simulink library "solar_panel_power_lib"  (R2016b)
settings: Solver=VariableStepAuto  StartTime=0.0  StopTime=10.0  RelTol=1e-3
undefined symbols (not defined in the file or in its folder): sim_params
libraries: aerolibutil x1
settings Model: Creator=taylorreynolds  LastModifiedBy=Taylor

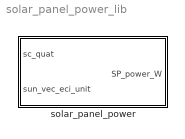
== system solar_panel_power_lib ==
  solar_panel_power : Subsystem

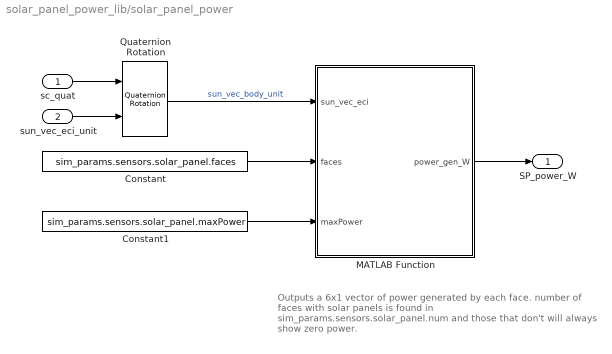
== system solar_panel_power_lib/solar_panel_power ==
  note: Outputs a 6x1 vector of power generated by each face.
      | number of faces with solar panels is found in
      | sim_params.sensors.solar_panel.num
      | and those that don't will always show zero power.
  sc_quat : Inport
  sun_vec_eci_unit : Inport  Port=2
  Constant : Constant  Value=sim_params.sensors.solar_panel.faces
  Constant1 : Constant  Value=sim_params.sensors.solar_panel.maxPower
  MATLAB Function : MATLAB Function  TreatAsAtomicUnit=on
  Quaternion Rotation : aerolibutil/Quaternion Rotation
  SP_power_W : Outport
  wires:
  sun_vec_eci_unit/1 -> Quaternion Rotation/2
  sc_quat/1 -> Quaternion Rotation/1
  MATLAB Function/1(power_gen_W) -> SP_power_W/1
  Quaternion Rotation/1 -> MATLAB Function/1(sun_vec_eci)  "sun_vec_body_unit"
  Constant/1 -> MATLAB Function/2(faces)
  Constant1/1 -> MATLAB Function/3(maxPower)

== matlab function solar_panel_power_lib/solar_panel_power/MATLAB Function ==
  data: sun_vec_eci input; power_gen_W output; faces input; maxPower input
function power_gen_W = get_power_gen(sun_vec_eci,faces,maxPower)
%GET_POWER_GEN
% 
% get_power_gen(sun_vec_eci,faces,maxPower) computes the total power being
% generated by the solar panels located on each of 'faces'. Assumes power
% generation is proportional to the square of the cosine of the incidence 
% angle to the sun, and can generate a maximum of 'maxPower' for each face.
%
% Assumes there are solar panels on all 6 sides of cuboid s/c, but fewer
% faces can be modeled by setting the maxPower of those faces to zero.
% ORDER OF FACES: [ +x, -x, +y, -y, +z, -z ]
%
% T. Reynolds -- 09.20.18
%#codegen

power_gen_W = zeros(6,1);

for i = 1:6
   face = faces(:,i);
   maxW = maxPower(i);
   
   sdotf = dot(face,sun_vec_eci);
   cinc  = saturate(sdotf);
   cinc2 = cinc * cinc;
   
   % compute power generated on ith face
   power_gen_W(i) = maxW * cinc2;
end

end

function y = saturate(x)
    if( x < 0 )
        y = 0.0;
    elseif( x > 1 )
        y = 1.0;
    else
        y = x;
    end
end
